simulink model "PIDresonant"  (R2021a)
settings: Solver=ode45  StartTime=0.0  StopTime=5  FixedStep=0.0001  RelTol=1e-3
values from neighbouring files (symbols this model uses):
  Beq = 1.067548701517996e-06    (= 1.06754870152e-06)    [load_params_resonantLoad.m]
  den_B = [mld.Jb, mld.Bb]    [load_params_resonantLoad.m]
  Jeq = mot.J + mld.Jh/gbox.N^2    [load_params_resonantLoad.m]
  Kd = Kp*Td    [PIDresonant_code.m]
  Ki = Kp/Ti    [PIDresonant_code.m]
  Kp = delta_K * cos(delta_phi)    [PIDresonant_code.m]
  Kw = 5/t_sett_5    (= 5.88235294118)    [PIDresonant_code.m]
  rads2rpm = 60/2/pi    (= 9.54929658551)    [load_params_resonantLoad.m]
  Req = mot.R + sens.curr.Rs    [load_params_resonantLoad.m]
  tau_sf = 0.012480599355650    (= 0.0124805993556)    [load_params_resonantLoad.m]
  Tl = 1/(beta*w_gc_star)    [PIDresonant_code.m]
  Ts = 0.001    [PIDresonant_code.m]    (also in SS_LRQ_commonStart.m)
undefined symbols (not defined in the file or in its folder): daq, DiscIntNeverNeededParam, drv, gbox, mld, mot, sens
libraries: simulink x2
settings Model: Creator=giorgiadisaro  LastModifiedBy=utente-A
settings SolverCC: AlgebraicLoopSolver=TrustRegion
settings DebuggingCC: SFMachineParentedDataDiag=warning

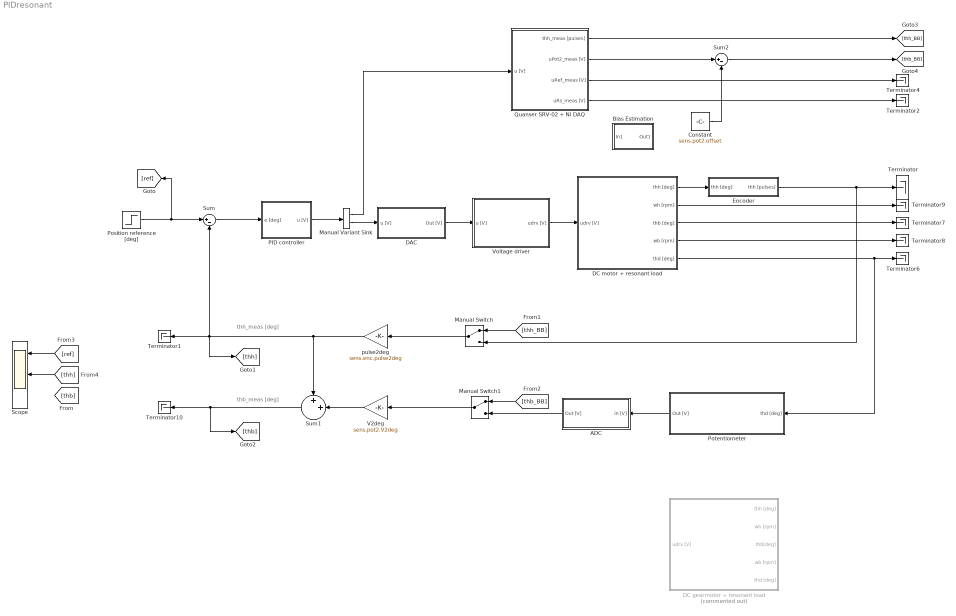
== system PIDresonant ==
  note: thh_meas [deg]
  note: thb_meas [deg]
  ADC : Subsystem
  Bias Estimation : Subsystem
  Constant : Constant  Value=sens.pot2.offset
  DAC : Subsystem
  DC gearmotor + resonant load : Subsystem  Commented=on
  DC motor + resonant load : Subsystem
  Encoder : Subsystem
  Manual Variant Sink : simulink/Signal Routing/Manual Variant Sink  NumChoices=2  LabelModeActiveChoice=V_1
  Manual Switch : ManualSwitch
  Manual Switch1 : ManualSwitch
  PID controller : Subsystem
  Position reference [deg] : Step  After=50  SampleTime=0
  Potentiometer : Subsystem
  Quanser SRV-02 + NI DAQ : Subsystem  mask(Quanser SRV-02 (with resonant load) + NI DAQ){Ts=0.001, fricType=Coulomb + viscous, lockShaft=off, beamInitPos=10}
      mask prompts: Ts "NI DAQ Sample Time:"; fricType "Friction model"; lockShaft "Lock motor shaft"; beamInitPos "Beam initial position [deg]:"
      mask help: Quanser SRV-02 (with resonant load) + NI DAQ model.
      mask init:
      | %%
      | % Riccardo Antonello (riccardo.antonello@unipd.it)
      | %
      | % April 28, 2020
      | %
      | % Dept. of Information Engineering, University of Padova
      | %
      | 
      | %%  Conversion gains
      | deg2rad = pi/180;                   %   [deg]   -> [rad]
      | rad2deg = 180/pi;                   %   [rad]   -> [deg]
      | 
      | 
      | %%  Sensors data
      | 
      | %   shunt resistor
      | sens.curr.Rs = 0.5;   
      | 
      | %   Hewlett-Packard HEDS-5540#A06 optical encoder
      | sens.enc.ppr = 500*4;                                                   %   pulses per rotation
      | sens.enc.pulse2deg = 360/sens.enc.ppr;                                  %   [pulses] -> [deg]
      | sens.enc.pulse2rad = 2*pi/sens.enc.ppr;                                 %   [pulses] -> [rad]
      | sens.enc.deg2pulse = sens.enc.ppr/360;                                  %   [deg] -> [pulses]
      | sens.enc.rad2pulse = sens.enc.ppr/2/pi;                                 %   [rad] -> [pulses]
      | 
      | %   potentiometer 2 (Spectrol 357-0-0-103) - installed on hub
      | sens.pot2.range.R      = 10e3;                                          %   ohmic value range 
      | sens.pot2.range.V      = 5;                                             %   voltage range
      | sens.pot2.range.th_deg = 340;                                           %   angle range [deg]
      | sens.pot2.range.th     = sens.pot2.range.th_deg * deg2rad;              %   angle range [rad]                           
      | sens.pot2.deg2V        = sens.pot2.range.V / sens.pot2.range.th_deg;    %   sensitivity [V/deg]
      | sens.pot2.rad2V        = sens.pot2.range.V / sens.pot2.range.th;        %   sensitivity [V/rad]
      | sens.pot2.V2deg        = 1/sens.pot2.deg2V;                             %   conversion gain [V] -> [deg]
      | sens.pot2.V2rad        = 1/sens.pot2.rad2V;                             %   conversion gain [V] -> [rad]
      | sens.pot2.noise.var    = 3.5e-7;                                        %   out noise variance [V^2]
      | 
      | 
      | %%  Data acquisition board (daq) data
      | 
      | %   NI PCI-6221 DAC data
      | daq.dac.bits = 16;                                  %   resolution (bits)
      | daq.dac.fs   = 10;                                  %   full scale 
      | daq.dac.q    = 2*daq.dac.fs/(2^daq.dac.bits-1);     %	quantization
      | 
      | %   NI PCI-6221 ADC data
      | daq.adc.bits = 16;                                  %   resolution (bits)
      | daq.adc.fs   = 10;                                  %   full scale (as set in SLDRT Analog Input block)
      | daq.adc.q    = 2*daq.adc.fs/(2^daq.adc.bits-1);     %   quantization   
      | 
      | 
      | %%  Set beam initial position
      | % SRV02Handle = find_system(gcb, ...
      | %     'LookUnderMasks', 'on', ...
      | %     'FindAll', 'on', ...
      | %     'FollowLinks', 'on', ...
      | %     'SearchDepth', '1', ...
      | %     'BlockType', 'ModelReference', ...
      | %     'Name', 'Quanser SRV-02');
      | %
      | % %get_param(SRV02Handle, 'InstanceParameters')
      | % InstanceParams = get_param(SRV02Handle, 'InstanceParameters');
      | % for k = 1:length(InstanceParams)
      | %     if strcmp(InstanceParams(k).Name, 'thb0')
      | %         if lockShaft
      | %             InstanceParams(k).Value = sprintf('%f', beamInitPos);
      | %         else
      | %             InstanceParams(k).Value = sprintf('%f', 0);    
      | %         end
      | %         set_param(SRV02Handle, 'InstanceParameters', InstanceParams);
      | %         break;
      | %     end
      | % end
      | 
      | if lockShaft
      |     thb0 = beamInitPos;
      | else
      |     thb0 = 0;    
      | end
      | 
      | 
      | %%  Mask initialization
      | if lockShaft
      |     
      |     %   find Inport handle
      |     InPortHandle = find_system(gcb, ...
      |         'LookUnderMasks', 'on', ...
      |         'FindAll', 'on', ...
      |         'FollowLinks', 'on', ...
      |         'SearchDepth', '1', ...
      |         'BlockType', 'Inport', ...
      |         'Name', 'u [V]');
      |     
      |     if ~isempty(InPortHandle)
      |     
      |         %   find DAC handle
      |         DACHandle = find_system(gcb, ...
      |             'LookUnderMasks', 'on', ...
      |             'FindAll', 'on', ...
      |             'FollowLinks', 'on', ...
      |             'SearchDepth', '1', ...
      |             'BlockType', 'SubSystem', ...
      |             'Name', 'DAC');  
      | 
      |         %   remove Inport output connection   
      |         InportConn = get_param(InPortHandle, 'PortConnectivity');
      |         delete_line(gcb, InportConn.Position);
      | 
      |         %   remove Inport block
      |         delete_block(InPortHandle);
      | 
      |         %   add Constant block
      |         ConstantHandle = add_block( ...
      |             'simulink/Sources/Constant', [gcb, '/u [V]'], ...
      |             'Position', [20   -37    50   -23], ...
      |             'Value', '0');
      | 
      |         %   connect Constant to DAC block
      |         DACPortHandles = get_param(DACHandle, 'PortHandles');
      |         ConstantPortHandles = get_param(ConstantHandle, 'PortHandles');
      |         add_line(gcb, ConstantPortHandles.Outport(1), DACPortHandles.Inport(1));
      |     
      |     end
      |     
      | else
      |     
      |     %   find Constant handle
      |     ConstantHandle = find_system(gcb, ...
      |         'LookUnderMasks', 'on', ...
      |         'FindAll', 'on', ...
      |         'FollowLinks', 'on', ...
      |         'SearchDepth', '1', ...
      |         'BlockType', 'Constant', ...
      |         'Name', 'u [V]');
      |     
      |     if ~isempty(ConstantHandle)
      |     
      |         %   find DAC handle
      |         DACHandle = find_system(gcb, ...
      |             'LookUnderMasks', 'on', ...
      |             'FindAll', 'on', ...
      |             'FollowLinks', 'on', ...
      |             'SearchDepth', '1', ...
      |             'BlockType', 'SubSystem', ...
      |             'Name', 'DAC');  
      |  
      |         %   remove Constant output connection   
      |         ConstantConn = get_param(ConstantHandle, 'PortConnectivity');
      |         delete_line(gcb, ConstantConn.Position);
      | 
      |         %   remove Inport block
      |         delete_block(ConstantHandle);   
      | 
      |         %   add Inport block
      |         InportHandle = add_block( ...
      |             'simulink/Sources/In1', [gcb, '/u [V]'], ...
      |             'Position', [20   -37    50   -23], ...
      |             'Port', '1');
      | 
      |         %   connect Constant to DAC block
      |         DACPortHandles = get_param(DACHandle, 'PortHandles');
      |         InportPortHandles = get_param(InportHandle, 'PortHandles');
      |         add_line(gcb, InportPortHandles.Outport(1), DACPortHandles.Inport(1));
      |     
      |      end
      |     
      | end
      mask Help:
      | Riccardo Antonello (antonello@dei.unipd.it)
      | 
      | April 28, 2020
      | 
      | Dept. of Information Engineering, University of Padova
      mask TypeOptions fricType: Coulomb + viscous | Karnopp
      mask Callback lockShaft:
      | %   get status of check box
      | lockShaft = get_param(gcb, 'lockShaft');
      | 
      | %   get current value of MaskVisibilities property
      | maskVisibilities = get_param(gcb, 'MaskVisibilities');
      | 
      | %   set visibility of the dialog box element
      | if strcmp(lockShaft, 'on')
      |     maskVisibilities{4} = 'on';
      | else
      |     maskVisibilities{4} = 'off';
      | end
      | 
      | % Set the 'MaskVisibilities' property for each parameter in mask
      | set_param( gcb, 'MaskVisibilities', maskVisibilities);
  Scope : Scope  NumInputPorts=3
  Sum : Sum  Inputs=|+-
  Sum1 : Sum  Inputs=++|
  Sum2 : Sum  Inputs=|+-
  Terminator{,1..2,4,6..10} (9 alike) : Terminator
  V2deg : Gain  Gain=sens.pot2.V2deg
  Voltage driver : Subsystem
  pulse2deg : Gain  Gain=sens.enc.pulse2deg
  wires:
  Manual Variant Sink/2 -> DAC/1(u [V])
  Manual Switch/1 -> pulse2deg/1
  DAC/1(Out [V]) -> Voltage driver/1(u [V])
  Sum/1 -> PID controller/1(e [deg])
  pulse2deg/1 -> Sum1/1, [thh], Sum/2, Terminator1/1
  PID controller/1(u [V]) -> Manual Variant Sink/1
  Position reference [deg]/1 -> [ref], Sum/1
  Encoder/1(thh [pulses]) -> Manual Switch/2, Terminator/1
  Manual Variant Sink/1 -> Quanser SRV-02 + NI DAQ/1(u [V])
  Quanser SRV-02 + NI DAQ/1(thh_meas [pulses]) -> [thh_BB]
  Quanser SRV-02 + NI DAQ/3(uRef_meas [V]) -> Terminator4/1
  Quanser SRV-02 + NI DAQ/4(uRs_meas [V]) -> Terminator2/1
  Potentiometer/1(Out [V]) -> ADC/1(in [V])
  V2deg/1 -> Sum1/2
  Sum1/1 -> [thb], Terminator10/1
  Quanser SRV-02 + NI DAQ/2(uPot2_meas [V]) -> Sum2/1
  Sum2/1 -> [thb_BB]
  Manual Switch1/1 -> V2deg/1
  [thh_BB] -> Manual Switch/1
  [thb_BB] -> Manual Switch1/1
  ADC/1(Out [V]) -> Manual Switch1/2
  [thh] -> Scope/2
  [ref] -> Scope/1
  Constant/1 -> Sum2/2
  DC motor + resonant load/1("thh [deg] ") -> Encoder/1("thh [deg] ")
  DC motor + resonant load/2(wh [rpm]) -> Terminator9/1
  DC motor + resonant load/3(thb [deg]) -> Terminator7/1
  DC motor + resonant load/4(wb [rpm]) -> Terminator8/1
  DC motor + resonant load/5(thd [deg]) -> Potentiometer/1(thd [deg]), Terminator6/1
  Voltage driver/1(udrv [V]) -> DC motor + resonant load/1(udrv [V])

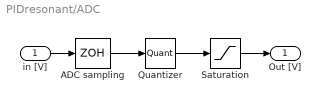
== system PIDresonant/ADC ==
  in [V] : Inport
  ADC sampling : ZeroOrderHold  SampleTime=Ts
  Quantizer : Quantizer  QuantizationInterval=daq.adc.q
  Saturation : Saturate  UpperLimit=daq.adc.fs  LowerLimit=-daq.adc.fs
  Out [V] : Outport
  wires:
  in [V]/1 -> ADC sampling/1
  ADC sampling/1 -> Quantizer/1
  Quantizer/1 -> Saturation/1
  Saturation/1 -> Out [V]/1

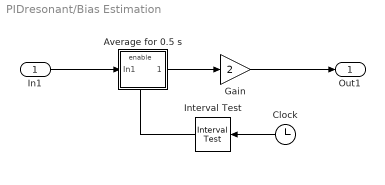
== system PIDresonant/Bias Estimation ==
  In1 : Inport
  Average for 0.5 s : Subsystem
  Clock : Clock
  Gain : Gain  Gain=2
  Interval Test : simulink/Logic and Bit Operations/Interval Test  IntervalClosedRight=on  uplimit=0.7  IntervalClosedLeft=on  lowlimit=0.2  OutDataTypeStr=boolean
  Out1 : Outport
  wires:
  Gain/1 -> Out1/1
  Average for 0.5 s/1(Out1) -> Gain/1
  Clock/1 -> Interval Test/1
  In1/1 -> Average for 0.5 s/1(In1)
  Interval Test/1 -> Average for 0.5 s/Enable

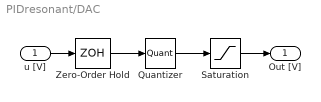
== system PIDresonant/DAC ==
  u [V] : Inport
  Quantizer : Quantizer  QuantizationInterval=daq.dac.q
  Saturation : Saturate  UpperLimit=daq.dac.fs  LowerLimit=-daq.dac.fs
  Zero-Order Hold : ZeroOrderHold  SampleTime=Ts
  Out [V] : Outport
  wires:
  u [V]/1 -> Zero-Order Hold/1
  Zero-Order Hold/1 -> Quantizer/1
  Quantizer/1 -> Saturation/1
  Saturation/1 -> Out [V]/1

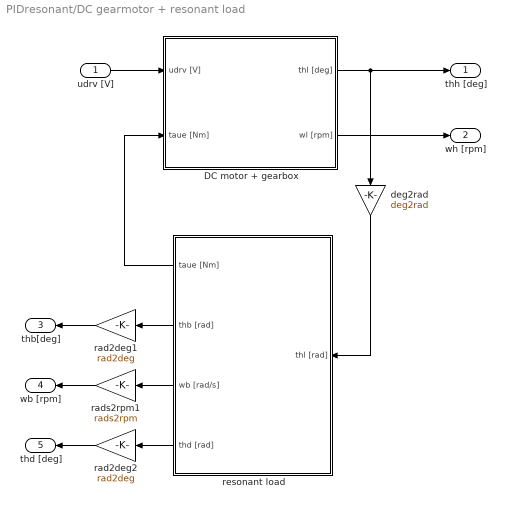
== system PIDresonant/DC gearmotor + resonant load ==
  udrv [V] : Inport
  DC motor + gearbox : Subsystem
  deg2rad : Gain  Gain=deg2rad
  rad2deg1 : Gain  Gain=rad2deg
  rad2deg2 : Gain  Gain=rad2deg
  rads2rpm1 : Gain  Gain=rads2rpm
  resonant load : Subsystem
  thh [deg] : Outport
  wh [rpm] : Outport  Port=2
  thb[deg] : Outport  Port=3
  wb [rpm] : Outport  Port=4
  thd [deg] : Outport  Port=5
  wires:
  udrv [V]/1 -> DC motor + gearbox/1(udrv [V])
  DC motor + gearbox/2(wl [rpm]) -> wh [rpm]/1
  resonant load/1(taue [Nm]) -> DC motor + gearbox/2(taue [Nm])
  resonant load/2(thb [rad]) -> rad2deg1/1
  rads2rpm1/1 -> wb [rpm]/1
  resonant load/3(wb [rad/s]) -> rads2rpm1/1
  rad2deg2/1 -> thd [deg]/1
  resonant load/4(thd [rad]) -> rad2deg2/1
  rad2deg1/1 -> thb[deg]/1
  DC motor + gearbox/1("thl [deg] ") -> thh [deg]/1, deg2rad/1
  deg2rad/1 -> resonant load/1("thl [rad] ")

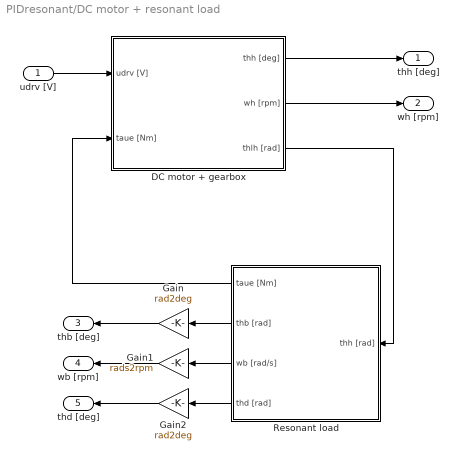
== system PIDresonant/DC motor + resonant load ==
  udrv [V] : Inport
  DC motor + gearbox : Subsystem
  Gain : Gain  Gain=rad2deg
  Gain1 : Gain  Gain=rads2rpm
  Gain2 : Gain  Gain=rad2deg
  Resonant load : Subsystem
  "thh [deg] " : Outport
  wh [rpm] : Outport  Port=2
  thb [deg] : Outport  Port=3
  wb [rpm] : Outport  Port=4
  thd [deg] : Outport  Port=5
  wires:
  DC motor + gearbox/3(thlh [rad]) -> Resonant load/1(thh [rad])
  DC motor + gearbox/1("thh [deg] ") -> "thh [deg] "/1
  Resonant load/1(taue [Nm]) -> DC motor + gearbox/2(taue [Nm])
  udrv [V]/1 -> DC motor + gearbox/1(udrv [V])
  DC motor + gearbox/2(wh [rpm]) -> wh [rpm]/1
  Resonant load/2(thb [rad]) -> Gain/1
  Gain/1 -> thb [deg]/1
  Gain1/1 -> wb [rpm]/1
  Resonant load/3(wb [rad/s]) -> Gain1/1
  Resonant load/4(thd [rad]) -> Gain2/1
  Gain2/1 -> thd [deg]/1

== system PIDresonant/Encoder ==
  "thh [deg] " : Inport
  Gain : Gain  Gain=2000/360
  Quantizer : Quantizer  QuantizationInterval=360/(500*4)
  Zero-Order Hold : ZeroOrderHold  SampleTime=Ts
  thh [pulses] : Outport
  wires:
  "thh [deg] "/1 -> Zero-Order Hold/1
  Zero-Order Hold/1 -> Quantizer/1
  Quantizer/1 -> Gain/1
  Gain/1 -> thh [pulses]/1

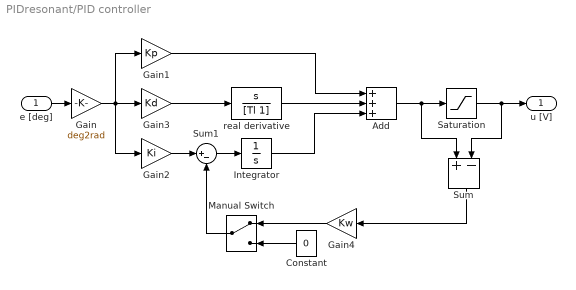
== system PIDresonant/PID controller ==
  e [deg] : Inport
  Add : Sum  Inputs=+++
  Constant : Constant  Value=0
  Gain : Gain  Gain=deg2rad
  Gain1 : Gain  Gain=Kp
  Gain2 : Gain  Gain=Ki
  Gain3 : Gain  Gain=Kd
  Gain4 : Gain  Gain=Kw
  Integrator : Integrator
  Manual Switch : ManualSwitch
  Saturation : Saturate  UpperLimit=10  LowerLimit=-10
  Sum : Sum  Inputs=+-
  Sum1 : Sum  Inputs=|+-
  real derivative : TransferFcn  Numerator=[1 0]  Denominator=[Tl 1]
  u [V] : Outport
  wires:
  Gain/1 -> Gain3/1, Gain1/1, Gain2/1
  Gain1/1 -> Add/1
  e [deg]/1 -> Gain/1
  Add/1 -> Sum/1, Saturation/1
  Saturation/1 -> Sum/2, u [V]/1
  Gain3/1 -> real derivative/1
  Sum1/1 -> Integrator/1
  Gain2/1 -> Sum1/1
  Sum/1 -> Gain4/1
  Gain4/1 -> Manual Switch/1
  Manual Switch/1 -> Sum1/2
  Constant/1 -> Manual Switch/2
  real derivative/1 -> Add/2
  Integrator/1 -> Add/3

== system PIDresonant/Potentiometer ==
  thd [deg] : Inport
  Gain : Gain  Gain=sens.pot2.deg2V
  Sum : Sum  Inputs=|++
  sensor output noise [V] : RandomNumber  Variance=sens.pot2.noise.var  SampleTime=Ts
  Out [V] : Outport
  wires:
  thd [deg]/1 -> Gain/1
  Gain/1 -> Sum/1
  Sum/1 -> Out [V]/1
  sensor output noise [V]/1 -> Sum/2

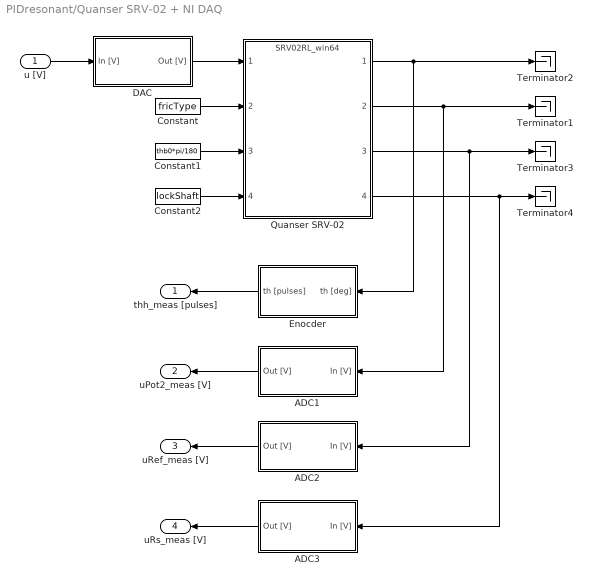
== system PIDresonant/Quanser SRV-02 + NI DAQ ==
  u [V] : Inport
  ADC1 : Subsystem
  ADC2 : Subsystem
  ADC3 : Subsystem
  Constant : Constant  Value=fricType
  Constant1 : Constant  Value=thb0*pi/180  SampleTime=Inf
  Constant2 : Constant  Value=lockShaft  SampleTime=Inf
  DAC : Subsystem
  Enocder : Subsystem
  Quanser SRV-02 : ModelReference  ModelNameDialog=SRV02RL_win64.slxp  ModelReferenceVersion=1.76  CopyOfModelProtected=on
  Terminator{1..4} (4 alike) : Terminator
  thh_meas [pulses] : Outport
  uPot2_meas [V] : Outport  Port=2
  uRef_meas [V] : Outport  Port=3
  uRs_meas [V] : Outport  Port=4
  wires:
  Enocder/1(th [pulses]) -> thh_meas [pulses]/1
  ADC3/1(Out [V]) -> uRs_meas [V]/1
  DAC/1(Out [V]) -> Quanser SRV-02/1
  Quanser SRV-02/2 -> ADC1/1(In [V]), Terminator1/1
  Quanser SRV-02/1 -> Terminator2/1, Enocder/1(th [deg])
  Constant/1 -> Quanser SRV-02/2
  Quanser SRV-02/3 -> ADC2/1(In [V]), Terminator3/1
  ADC1/1(Out [V]) -> uPot2_meas [V]/1
  Constant1/1 -> Quanser SRV-02/3
  Constant2/1 -> Quanser SRV-02/4
  Quanser SRV-02/4 -> ADC3/1(In [V]), Terminator4/1
  ADC2/1(Out [V]) -> uRef_meas [V]/1
  u [V]/1 -> DAC/1(In [V])

== system PIDresonant/Voltage driver ==
  u [V] : Inport
  Saturation : Saturate  UpperLimit=12  LowerLimit=-12
  Transfer Fcn : TransferFcn  Numerator=[drv.dcgain]  Denominator=[drv.Tc 1]
  udrv [V] : Outport
  wires:
  u [V]/1 -> Transfer Fcn/1
  Transfer Fcn/1 -> Saturation/1
  Saturation/1 -> udrv [V]/1

== system PIDresonant/Bias Estimation/Average for 0.5 s ==
  In1 : Inport
  Enable : EnablePort
  Discrete-Time Integrator : DiscreteIntegrator  SampleTime=Ts  ICPrevOutput=DiscIntNeverNeededParam  ICPrevScaledInput=DiscIntNeverNeededParam
  Out1 : Outport
  wires:
  Discrete-Time Integrator/1 -> Out1/1
  In1/1 -> Discrete-Time Integrator/1

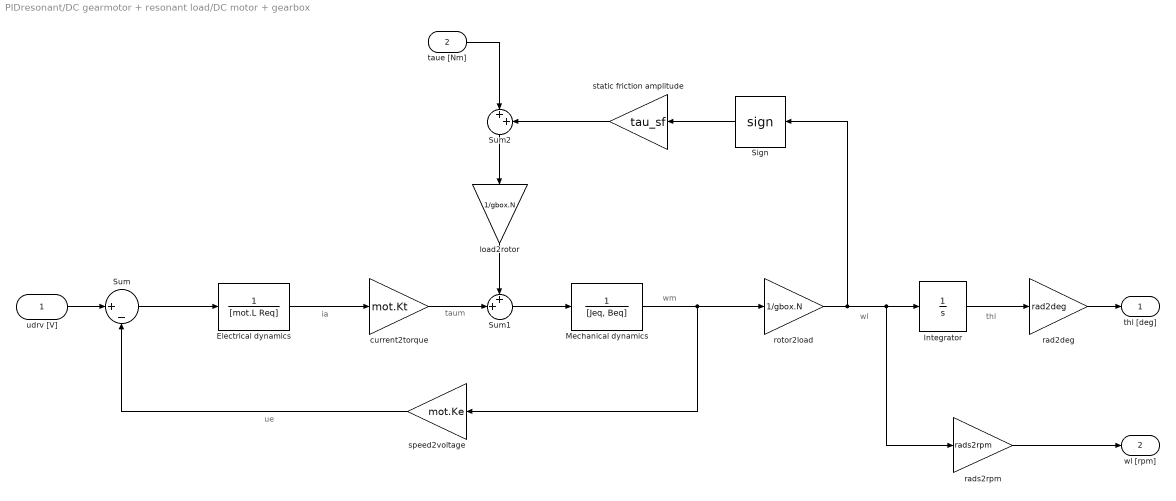
== system PIDresonant/DC gearmotor + resonant load/DC motor + gearbox ==
  note: thl
  note: wl
  note: wm
  note: ue
  note: taum
  note: ia
  udrv [V] : Inport
  taue [Nm] : Inport  Port=2
  Electrical dynamics : TransferFcn  Denominator=[mot.L Req]
  Integrator : Integrator
  Mechanical dynamics : TransferFcn  Denominator=[Jeq, Beq]
  Sign : Signum  ZeroCross=off
  Sum : Sum  Inputs=|+-
  Sum1 : Sum  Inputs=++|
  Sum2 : Sum  Inputs=|++
  current2torque : Gain  Gain=mot.Kt
  load2rotor : Gain  Gain=1/gbox.N
  rad2deg : Gain  Gain=rad2deg
  rads2rpm : Gain  Gain=rads2rpm
  rotor2load : Gain  Gain=1/gbox.N
  speed2voltage : Gain  Gain=mot.Ke
  static friction amplitude : Gain  Gain=tau_sf
  "thl [deg] " : Outport
  wl [rpm] : Outport  Port=2
  wires:
  udrv [V]/1 -> Sum/1
  Electrical dynamics/1 -> current2torque/1
  Sign/1 -> static friction amplitude/1
  speed2voltage/1 -> Sum/2
  rad2deg/1 -> "thl [deg] "/1
  Sum1/1 -> Mechanical dynamics/1
  Mechanical dynamics/1 -> rotor2load/1, speed2voltage/1
  rads2rpm/1 -> wl [rpm]/1
  Sum/1 -> Electrical dynamics/1
  rotor2load/1 -> Sign/1, rads2rpm/1, Integrator/1
  Integrator/1 -> rad2deg/1
  current2torque/1 -> Sum1/2
  load2rotor/1 -> Sum1/1
  static friction amplitude/1 -> Sum2/2
  Sum2/1 -> load2rotor/1
  taue [Nm]/1 -> Sum2/1

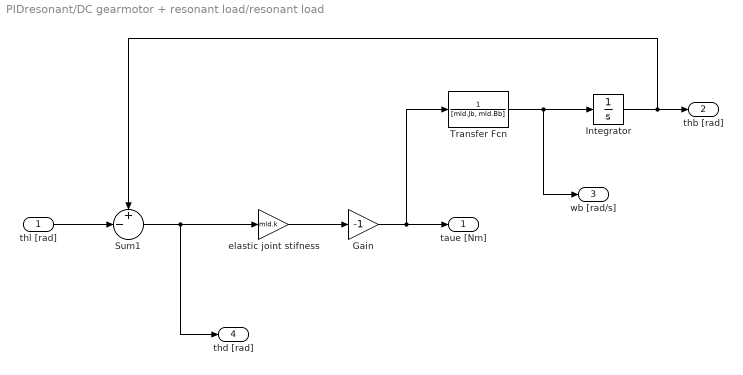
== system PIDresonant/DC gearmotor + resonant load/resonant load ==
  "thl [rad] " : Inport
  Gain : Gain  Gain=-1
  Integrator : Integrator
  Sum1 : Sum  Inputs=+-|
  Transfer Fcn : TransferFcn  Denominator=[mld.Jb, mld.Bb]
  elastic joint stifness : Gain  Gain=mld.k
  taue [Nm] : Outport
  thb [rad] : Outport  Port=2
  wb [rad/s] : Outport  Port=3
  thd [rad] : Outport  Port=4
  wires:
  "thl [rad] "/1 -> Sum1/2
  Sum1/1 -> elastic joint stifness/1, thd [rad]/1
  elastic joint stifness/1 -> Gain/1
  Gain/1 -> taue [Nm]/1, Transfer Fcn/1
  Transfer Fcn/1 -> Integrator/1, wb [rad/s]/1
  Integrator/1 -> Sum1/1, thb [rad]/1

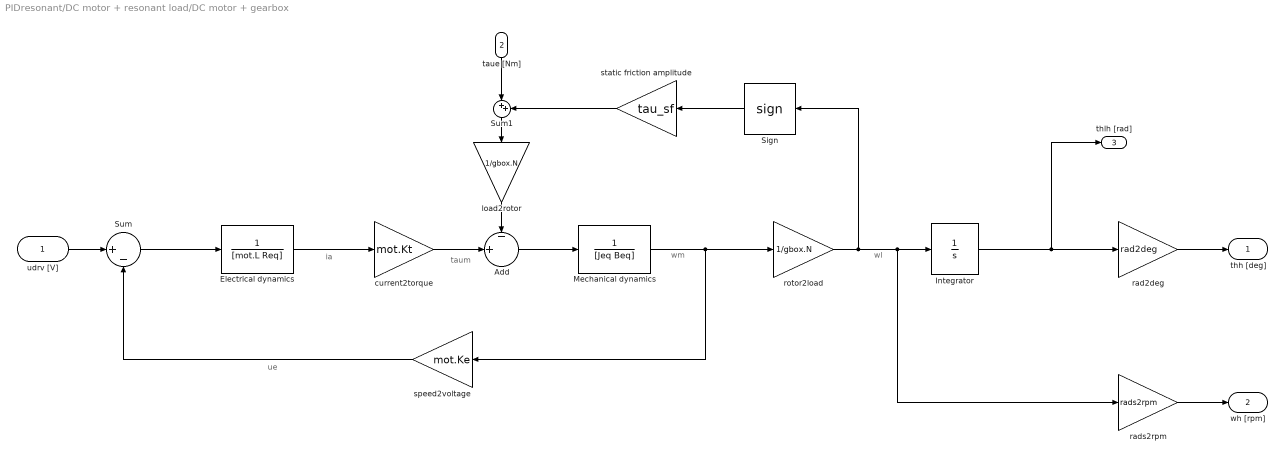
== system PIDresonant/DC motor + resonant load/DC motor + gearbox ==
  note: wl
  note: wm
  note: ue
  note: taum
  note: ia
  udrv [V] : Inport
  taue [Nm] : Inport  Port=2
  Add : Sum  Inputs=-|+||
  Electrical dynamics : TransferFcn  Denominator=[mot.L Req]
  Integrator : Integrator
  Mechanical dynamics : TransferFcn  Denominator=[Jeq Beq]
  Sign : Signum  ZeroCross=off
  Sum : Sum  Inputs=|+-
  Sum1 : Sum  Inputs=|++
  current2torque : Gain  Gain=mot.Kt
  load2rotor : Gain  Gain=1/gbox.N
  rad2deg : Gain  Gain=rad2deg
  rads2rpm : Gain  Gain=rads2rpm
  rotor2load : Gain  Gain=1/gbox.N
  speed2voltage : Gain  Gain=mot.Ke
  static friction amplitude : Gain  Gain=tau_sf
  "thh [deg] " : Outport
  wh [rpm] : Outport  Port=2
  thlh [rad] : Outport  Port=3
  wires:
  udrv [V]/1 -> Sum/1
  Electrical dynamics/1 -> current2torque/1
  current2torque/1 -> Add/2
  load2rotor/1 -> Add/1
  Sign/1 -> static friction amplitude/1
  speed2voltage/1 -> Sum/2
  rad2deg/1 -> "thh [deg] "/1
  Add/1 -> Mechanical dynamics/1
  Mechanical dynamics/1 -> speed2voltage/1, rotor2load/1
  rads2rpm/1 -> wh [rpm]/1
  Sum/1 -> Electrical dynamics/1
  rotor2load/1 -> Sign/1, rads2rpm/1, Integrator/1
  Integrator/1 -> rad2deg/1, thlh [rad]/1
  Sum1/1 -> load2rotor/1
  static friction amplitude/1 -> Sum1/2
  taue [Nm]/1 -> Sum1/1

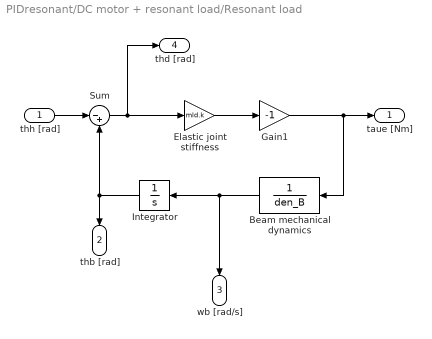
== system PIDresonant/DC motor + resonant load/Resonant load ==
  thh [rad] : Inport
  Beam mechanical dynamics : TransferFcn  Denominator=den_B
  Elastic joint stiffness : Gain  Gain=mld.k
  Gain1 : Gain  Gain=-1
  Integrator : Integrator
  Sum : Sum  Inputs=|-+
  taue [Nm] : Outport
  thb [rad] : Outport  Port=2
  wb [rad/s] : Outport  Port=3
  thd [rad] : Outport  Port=4
  wires:
  thh [rad]/1 -> Sum/1
  Integrator/1 -> thb [rad]/1, Sum/2
  Beam mechanical dynamics/1 -> Integrator/1, wb [rad/s]/1
  Sum/1 -> Elastic joint stiffness/1, thd [rad]/1
  Elastic joint stiffness/1 -> Gain1/1
  Gain1/1 -> Beam mechanical dynamics/1, taue [Nm]/1

== system PIDresonant/Quanser SRV-02 + NI DAQ/ADC1 ==
  In [V] : Inport
  ADC quantization : Quantizer  QuantizationInterval=daq.adc.q
  ADC sampling : ZeroOrderHold  SampleTime=Ts
  ADC saturation : Saturate  UpperLimit=daq.adc.fs  LowerLimit=-daq.adc.fs
  Out [V] : Outport
  wires:
  ADC saturation/1 -> Out [V]/1
  ADC sampling/1 -> ADC quantization/1
  In [V]/1 -> ADC sampling/1
  ADC quantization/1 -> ADC saturation/1

== system PIDresonant/Quanser SRV-02 + NI DAQ/ADC2 ==
  In [V] : Inport
  ADC quantization : Quantizer  QuantizationInterval=daq.adc.q
  ADC sampling : ZeroOrderHold  SampleTime=Ts
  ADC saturation : Saturate  UpperLimit=daq.adc.fs  LowerLimit=-daq.adc.fs
  Out [V] : Outport
  wires:
  ADC quantization/1 -> ADC saturation/1
  In [V]/1 -> ADC sampling/1
  ADC sampling/1 -> ADC quantization/1
  ADC saturation/1 -> Out [V]/1

== system PIDresonant/Quanser SRV-02 + NI DAQ/ADC3 ==
  In [V] : Inport
  Quantizer : Quantizer  QuantizationInterval=daq.adc.q
  Saturation : Saturate  UpperLimit=daq.adc.fs  LowerLimit=-daq.adc.fs
  Zero-Order Hold : ZeroOrderHold  SampleTime=Ts
  Out [V] : Outport
  wires:
  Saturation/1 -> Out [V]/1
  In [V]/1 -> Zero-Order Hold/1
  Quantizer/1 -> Saturation/1
  Zero-Order Hold/1 -> Quantizer/1

== system PIDresonant/Quanser SRV-02 + NI DAQ/DAC ==
  In [V] : Inport
  Quantizer : Quantizer  QuantizationInterval=daq.dac.q
  Saturation : Saturate  UpperLimit=daq.dac.fs  LowerLimit=-daq.dac.fs
  Zero-Order Hold : ZeroOrderHold  SampleTime=Ts
  Out [V] : Outport
  wires:
  Quantizer/1 -> Saturation/1
  In [V]/1 -> Zero-Order Hold/1
  Zero-Order Hold/1 -> Quantizer/1
  Saturation/1 -> Out [V]/1

== system PIDresonant/Quanser SRV-02 + NI DAQ/Enocder ==
  th [deg] : Inport
  Quantizer : Quantizer  QuantizationInterval=sens.enc.pulse2deg
  Zero-Order Hold : ZeroOrderHold  SampleTime=Ts
  deg2pulse : Gain  Gain=sens.enc.deg2pulse
  th [pulses] : Outport
  wires:
  Quantizer/1 -> deg2pulse/1
  th [deg]/1 -> Zero-Order Hold/1
  Zero-Order Hold/1 -> Quantizer/1
  deg2pulse/1 -> th [pulses]/1
